simulink model "Cherno_lab_4"  (Simulink 8.8)
settings: Solver=ode45  StartTime=0.0  StopTime=20  RelTol=1e-3  EnableMultiTasking=on
settings Model: Creator=student  LastModifiedBy=Admin
settings OptimizationCC: ExpressionDepthLimit=2147483647  InitFltsAndDblsToZero=on
settings DebuggingCC: SolverPrmCheckMsg=warning
settings GRTTargetCC: GeneratePreprocessorConditionals=Use local settings

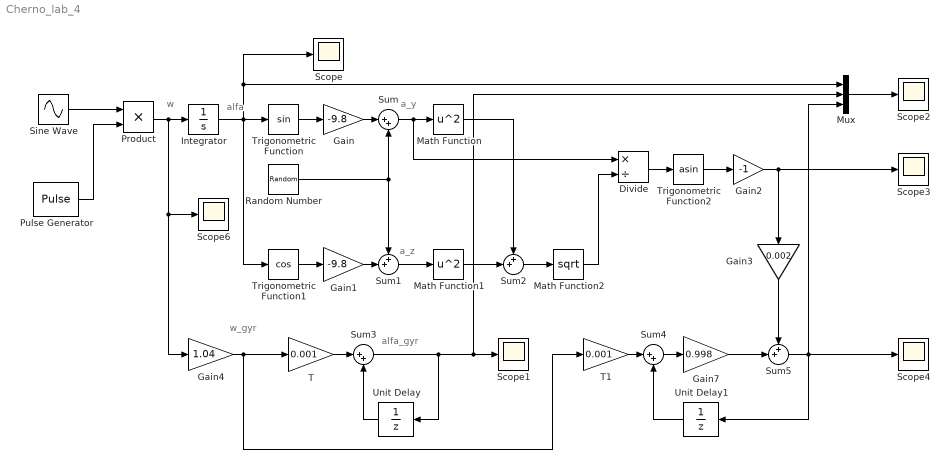
== system Cherno_lab_4 ==
  note: w_gyr
  note: alfa_gyr
  note: a_y
  note: a_z
  note: w
  note: alfa
  Divide : Product  Inputs=*/
  Gain : Gain  Gain=-9.8
  Gain1 : Gain  Gain=-9.8
  Gain2 : Gain  Gain=-1
  Gain3 : Gain  Gain=0.002
  Gain4 : Gain  Gain=1.04
  Gain7 : Gain  Gain=0.998
  Integrator : Integrator
  Math Function : Math  Operator=square  SaturateOnIntegerOverflow=on
  Math Function1 : Math  Operator=square  SaturateOnIntegerOverflow=on
  Math Function2 : Math  Operator=sqrt  SaturateOnIntegerOverflow=on
  Mux : Mux  Inputs=3
  Product : Product  RndMeth=Zero
  Pulse Generator : DiscretePulseGenerator  PulseType=Time based  Period=6  PulseWidth=33.3333333  PhaseDelay=4
  Random Number : RandomNumber  SampleTime=0
  Scope{,1..4,6} (6 alike) : Scope
  Sine Wave : Sin  Amplitude=pi/4  Frequency=2*pi*0.25  SampleTime=0
  Sum : Sum  Inputs=|++
  Sum1 : Sum  Inputs=++|
  Sum2 : Sum  Inputs=++|
  Sum3 : Sum  Inputs=|++
  Sum4 : Sum  Inputs=|++
  Sum5 : Sum  Inputs=++|
  T : Gain  Gain=0.001
  T1 : Gain  Gain=0.001
  Trigonometric Function : Trigonometry
  Trigonometric Function1 : Trigonometry  Operator=cos
  Trigonometric Function2 : Trigonometry  Operator=asin
  Unit Delay : UnitDelay  SampleTime=0.001
  Unit Delay1 : UnitDelay  SampleTime=0.001
  wires:
  Sine Wave/1 -> Product/1
  Pulse Generator/1 -> Product/2
  Product/1 -> Integrator/1, Gain4/1, Scope6/1
  Integrator/1 -> Trigonometric Function/1, Trigonometric Function1/1, Scope/1, Mux/1
  Trigonometric Function/1 -> Gain/1
  Gain/1 -> Sum/1
  Sum/1 -> Math Function/1, Divide/1
  Random Number/1 -> Sum/2, Sum1/1
  Trigonometric Function1/1 -> Gain1/1
  Gain1/1 -> Sum1/2
  Sum1/1 -> Math Function1/1
  Math Function/1 -> Sum2/1
  Math Function1/1 -> Sum2/2
  Sum2/1 -> Math Function2/1
  Math Function2/1 -> Divide/2
  Divide/1 -> Trigonometric Function2/1
  T/1 -> Sum3/1
  Unit Delay/1 -> Sum3/2
  T1/1 -> Sum4/1
  Unit Delay1/1 -> Sum4/2
  Gain3/1 -> Sum5/1
  Gain7/1 -> Sum5/2
  Sum4/1 -> Gain7/1
  Sum3/1 -> Unit Delay/1, Scope1/1, Mux/2
  Gain4/1 -> T/1, T1/1
  Trigonometric Function2/1 -> Gain2/1
  Gain2/1 -> Gain3/1, Scope3/1
  Sum5/1 -> Scope4/1, Mux/3, Unit Delay1/1
  Mux/1 -> Scope2/1
